simulink model "Lab_06_Task01"  (R2015a)
settings: Solver=ode45  StartTime=0.0  StopTime=10.0  RelTol=1e-3
settings Model: Creator=Amir  LastModifiedBy=Amir

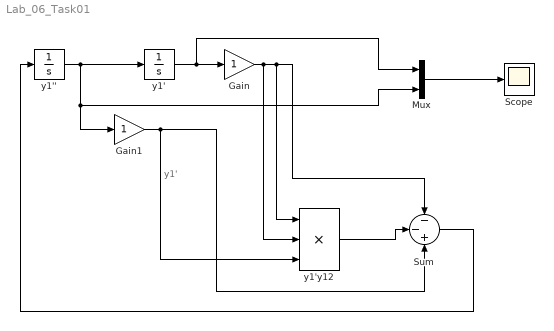
== system Lab_06_Task01 ==
  note: y1'
  Gain : Gain
  Gain1 : Gain
  Mux : Mux  Inputs=2
  Scope : Scope
  Sum : Sum  Inputs=--+
  y1' : Integrator
  y1'' : Integrator  InitialCondition=12
  y1'y12 : Product  Inputs=3
  wires:
  y1''/1 -> Mux/2, Gain1/1, y1'/1
  Mux/1 -> Scope/1
  Gain/1 -> y1'y12/2, y1'y12/1, Sum/1
  y1'y12/1 -> Sum/2
  Sum/1 -> y1''/1
  Gain1/1 -> y1'y12/3, Sum/3
  y1'/1 -> Mux/1, Gain/1
